simulink model "scar22"  (R2021a)
settings: Solver=ode23tb  StartTime=0.0  StopTime=.2  RelTol=1e-3
libraries: spsThreePhaseSeriesRLCLoadLib x17, spsThreePhasePISectionLineLib x16, spsThreePhaseTransformerTwoWindingsLib x14, spsThreePhaseVIMeasurementLib x11, simulink x6, exampleMicrogridLibrary x6, spsThreePhaseParallelRLCBranchLib x5, spsThreePhaseDynamicLoadLib x5, spsGroundLib x4, spsAC1AExcitationSystemLib x2, spsDieselMotorModel x2, spsSynchronousMachinepuStandardLib x2
(part 1 of 2)
settings Model: Creator=jlesage  LastModifiedBy=Administrator
settings SolverCC: AlgebraicLoopSolver=TrustRegion
settings DataIOCC: SaveFormat=Array  ReturnWorkspaceOutputs=off  DatasetSignalFormat=timetable
settings DebuggingCC: UnconnectedInputMsg=none  UnconnectedOutputMsg=none  UnconnectedLineMsg=none  SFMachineParentedDataDiag=warning  ArithmeticOperatorsInVariantConditions=warning
settings SFSimCC: SimUseLocalCustomCode=off  CustomCodeUndefinedFunction=UseInterfaceOnly
settings RTWCC: RTWUseLocalCustomCode=off

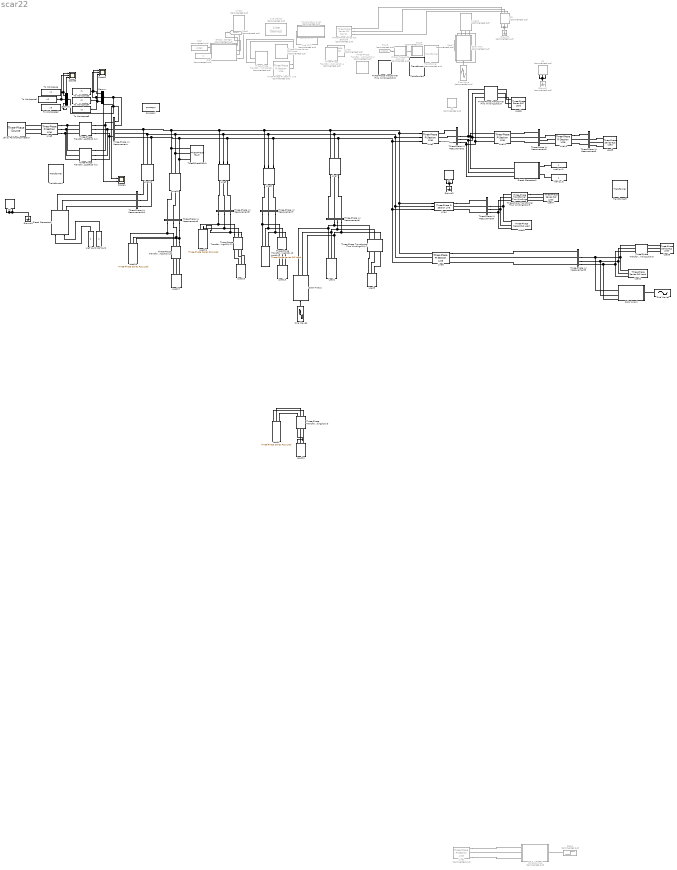
== system scar22 ==
  C1 : spsThreePhaseParallelRLCBranchLib/Three-Phase Parallel RLC Branch  Commented=on  LConnTagsString=A|B|C  RConnTagsString=A|B|C  BranchType=C  Resistance=1  Inductance=0.2e-2  Capacitance=550e-5  Measurements=None
      settings: SourceProductBaseCode=PS
  C2 : spsThreePhaseParallelRLCBranchLib/Three-Phase Parallel RLC Branch  Commented=on  LConnTagsString=A|B|C  RConnTagsString=A|B|C  BranchType=C  Resistance=1  Inductance=0.2e-2  Capacitance=550e-5  Measurements=None
      settings: SourceProductBaseCode=PS
  C3 : spsThreePhaseParallelRLCBranchLib/Three-Phase Parallel RLC Branch  Commented=on  LConnTagsString=A|B|C  RConnTagsString=A|B|C  BranchType=C  Resistance=1  Inductance=0.2e-2  Capacitance=550e-5  Measurements=None
      settings: SourceProductBaseCode=PS
  C4 : spsThreePhaseParallelRLCBranchLib/Three-Phase Parallel RLC Branch  LConnTagsString=A|B|C  RConnTagsString=A|B|C  BranchType=C  Resistance=1  Inductance=0.2e-2  Capacitance=1e6  Measurements=None
      settings: SourceProductBaseCode=PS
  C5 : spsThreePhaseParallelRLCBranchLib/Three-Phase Parallel RLC Branch  LConnTagsString=A|B|C  RConnTagsString=A|B|C  BranchType=R  Resistance=1e6  Inductance=0.2e-2  Capacitance=550e-5  Measurements=None
      settings: SourceProductBaseCode=PS
  Demux : Demux  Outputs=3
  Demux1 : Demux  Outputs=3
  Diesel Generator1 : Subsystem  mask(Diesel Generator (Simple)){Pn=3.5e6, Vn=10000, Fn=50, genType=PQ, PQ0=[0.05 0]}
      mask prompts: Pn "Generator Rated Power [W]"; Vn "Rated Voltage [V]"; Fn "Rated Frequency [Hz]"; genType "Load Flow Type"; PQ0 "Initial Power, [P0 Q0] [pu]"
      mask help:
      | The Diesel Generator block contains a synchronous generator, diesel governor and excitation system to represent the dynamics of a Genset. To inspect the model, look under the block mask (Ctrl + u).
      |
      | The inputs to the basic Diesel generator block are the desired speed reference (in pu) and the desired voltage reference (in pu). The output measurements are contained in a Simulink bus, which can be selected by using the Bus Selector block.
      |
      | Note: The initial generator power must be specified for use for Load Flow analysis.
      mask init:
      | % Extract Initial Active/Reactive Power
      | P0 = PQ0(1);
      | Q0 = PQ0(2);
      | 
      | % Select Load Flow Type
      | genBlock = [gcb '/Synchronous Machine'];
      | currentVals = get_param(genBlock,'MaskValues');
      | currentVals{31} = genType;
      | set_param(genBlock,'MaskValues',currentVals);
      | 
      | % Disable Option if Swing Generator Selected
      | currentEnables = get_param(gcb,'MaskEnables');
      | if strcmp(genType,'swing')
      |     currentEnables{5} = 'off';
      | else
      |     currentEnables{5} = 'on';
      | end
      | set_param(gcb,'MaskEnables',currentEnables);
      settings: AttributesFormatString=Rated Power: %<Pn> W
      mask TypeOptions genType: swing | PQ | PV
      mask Display: %image(imread('diesel.jpg'))
  Diesel Generator2 : Subsystem  mask(Diesel Generator (Simple)){Pn=7.6e6, Vn=10000, Fn=50, genType=PQ, PQ0=[0.05 0]}
      mask prompts: Pn "Generator Rated Power [W]"; Vn "Rated Voltage [V]"; Fn "Rated Frequency [Hz]"; genType "Load Flow Type"; PQ0 "Initial Power, [P0 Q0] [pu]"
      mask help:
      | The Diesel Generator block contains a synchronous generator, diesel governor and excitation system to represent the dynamics of a Genset. To inspect the model, look under the block mask (Ctrl + u).
      |
      | The inputs to the basic Diesel generator block are the desired speed reference (in pu) and the desired voltage reference (in pu). The output measurements are contained in a Simulink bus, which can be selected by using the Bus Selector block.
      |
      | Note: The initial generator power must be specified for use for Load Flow analysis.
      mask init: same as scar22/Diesel Generator1
      settings: AttributesFormatString=Rated Power: %<Pn> W
      mask TypeOptions genType: swing | PQ | PV
      mask Display: %image(imread('diesel.jpg'))
  Energy Storage : Subsystem  Commented=on  mask(Grid-connected Energy Storage (PQ Model)){Vn=5000, Fn=50, PnomkW=500, kWh_Rated=100, Efficiency=96, LimitVec=[90 10], RechargeSOC=11, Precharge=50, autoRecharge=off, Initial_kWh_pc=80, PQvec=[500e3 0]}
      mask prompts: Vn "Nominal L-L Voltage [Vrms]"; Fn "Nominal Frequency [Hz]"; PnomkW "Rated Power [kW]"; kWh_Rated "Rated Capacity [kWh]"; Efficiency "Overall System Efficiency [%]"; LimitVec "Upper/Lower Charge Limits [%]"; RechargeSOC "SOC to Recharge [%]"; Precharge "Recharge Rate [% of Rated Power]"; autoRecharge "Enable Auto-Recharge"; Initial_kWh_pc "Initial State-of-Charge [0-100%]"; PQvec "Initial Active/Reactive Cmds"
      mask help:
      | The energy storage block models a generic grid-connected energy storage system (ESS), most commonly a battery system. This is a system-level model that does not contain any power electronics, but is useful for load flow, phasor, and hybrid phasor-EMT simulations. The inputs to this block are the commanded active and reactive power of the ESS. The ESS is assumed to have four quadrent operation.
      |
      | For more detailed ESS models, consider the battery block in the Drives library. Consider using this PQ Model to perform load flow studies and switch to a more detailed model when full EMT studies or more advanced controls are required.
      |
      | Note: The initial active/reactive power commands must be specified for use for Load Flow analysis.
      mask init:
      | % Calculate Initial Conditions
      | Pnom = PnomkW*1e3;
      | P0 = -PQvec(1);  Q0 = -PQvec(2);
      | if abs(P0) > Pnom
      |     P0 = sign(P0)*Pnom;
      | end
      | 
      | % Calculate Q0 given Reactive Power Capability Curve
      | Qlim = sqrt(Pnom^2 - P0^2);
      | if Qlim > abs(Q0)
      |     Q0 = sign(Q0)*Qlim;
      | end
      | 
      | UpChrgLim = LimitVec(1);
      | LowChrgLim = LimitVec(2);
      | if Initial_kWh_pc > UpChrgLim && P0 < 0
      |     P0 = 0; Q0 = 0;
      | elseif Initial_kWh_pc < LowChrgLim && P0 > 0
      |     P0 = 0; Q0 = 0;
      | end
      mask DialogControl Container7 Prompt: Grid Connection Properties
      mask DialogControl Container11 Prompt: Charge/Discharge Controls
      mask DialogControl Container12 Prompt: Initial Conditions
  From3 : From  Commented=on  GotoTag=Vabc  TagVisibility=global
  Goto1 : Goto  Commented=on  GotoTag=battM  TagVisibility=global
  Goto2 : Goto  Commented=on  GotoTag=pvM  TagVisibility=global
  Ground1 : spsGroundLib/Ground  Commented=on  LConnTagsString=a
  Ground2 : spsGroundLib/Ground  LConnTagsString=a
  Ground3 : spsGroundLib/Ground  Commented=on  LConnTagsString=a
  Ground4 : spsGroundLib/Ground  LConnTagsString=a
  Line (PI)1 : exampleMicrogridLibrary/Line (PI)  Commented=on  gauge=500 Kcmil  Freq=60  Length_ft=50  Ratio=3
  Line (Series) : exampleMicrogridLibrary/Line (Series)  Commented=on  gauge=500 Kcmil  Length=50
  Line1 : spsThreePhasePISectionLineLib/Three-Phase PI Section Line  Commented=on  LConnTagsString=a|b|c  RConnTagsString=A|B|C  Length=1  Frequency=50  Resistances=[ 0.01273 0.3864]  Inductances="[ 0.9337e-3  4.1264e-3]"  Capacitances=[12.74e-9 7.751e-9]
  Line10 : spsThreePhasePISectionLineLib/Three-Phase PI Section Line  Commented=on  LConnTagsString=a|b|c  RConnTagsString=A|B|C  Length=1  Frequency=50  Resistances="[ 0.206  0.96 ]"  Inductances="[ 0.359e-3   1.178e-3 ]"  Capacitances="[0.254e-6  0.118e-6 ]"
  Line11 : spsThreePhasePISectionLineLib/Three-Phase PI Section Line  Commented=on  LConnTagsString=a|b|c  RConnTagsString=A|B|C  Length=1  Frequency=50  Resistances="[ 0.206  0.96 ]"  Inductances="[ 0.359e-3   1.178e-3 ]"  Capacitances="[0.254e-6  0.118e-6 ]"
  Line{2,4,6..9,12..15} (10 alike) : spsThreePhasePISectionLineLib/Three-Phase PI Section Line  LConnTagsString=a|b|c  RConnTagsString=A|B|C  Length=1  Frequency=50  Resistances="[ 0.206  0.96 ]"  Inductances="[ 0.359e-3   1.178e-3 ]"  Capacitances="[0.254e-6  0.118e-6 ]"
  Line3 : spsThreePhasePISectionLineLib/Three-Phase PI Section Line  Commented=on  LConnTagsString=a|b|c  RConnTagsString=A|B|C  Length=1  Frequency=50  Resistances="[ 0.206  0.96 ]"  Inductances="[ 0.359e-3   1.178e-3 ]"  Capacitances="[0.254e-6  0.118e-6 ]"
  Line5 : spsThreePhasePISectionLineLib/Three-Phase PI Section Line  LConnTagsString=a|b|c  RConnTagsString=A|B|C  Length=1  Frequency=50  Resistances=[ 0.01273 0.3864]  Inductances="[ 0.9337e-3  4.1264e-3]"  Capacitances=[12.74e-9 7.751e-9]
  Load{1..5,14,16,18} (8 alike) : spsThreePhaseSeriesRLCLoadLib/Three-Phase Series RLC Load  LConnTagsString=A|B|C  Configuration=Y (grounded)  NominalVoltage=10000  Vabc=[1e3 1e3 1e3]  Vabcp=[1e3 1e3 1e3]  NominalFrequency=50  UnbalancedPower=off  ActivePower=500e3  InductivePower=0  CapacitivePower=0  Pabc=[10e3 9e3 11e3]  QLabc=[100 90 110]  QCabc=[100 90 110]  Pabcp=[10e3 9e3 11e3]  QLabcp=[100 90 110]  QCabcp=[100 90 110]  Measurements=None  LoadType=constant Z
      settings: AttributesFormatString=P = %<ActivePower> W
  Load{6..10,13,15,17} (8 alike) : spsThreePhaseSeriesRLCLoadLib/Three-Phase Series RLC Load  LConnTagsString=A|B|C  Configuration=Y (grounded)  NominalVoltage=400  Vabc=[1e3 1e3 1e3]  Vabcp=[1e3 1e3 1e3]  NominalFrequency=50  UnbalancedPower=off  ActivePower=500e3  InductivePower=0  CapacitivePower=0  Pabc=[10e3 9e3 11e3]  QLabc=[100 90 110]  QCabc=[100 90 110]  Pabcp=[10e3 9e3 11e3]  QLabcp=[100 90 110]  QCabcp=[100 90 110]  Measurements=None  LoadType=constant Z
      settings: AttributesFormatString=P = %<ActivePower> W
  Phasor Sequence Analyzer : Subsystem  Commented=on
  Pref : Constant  Commented=on  Value=100e3
  Qref : Constant  Commented=on  Value=0
  Scope : Subsystem  Commented=on
  Scope1 : Scope  NumInputPorts=2
  Scope2 : Scope  NumInputPorts=3
  Scope3 : Scope  NumInputPorts=3
  Sine Wave : Sin  Commented=on  Amplitude=200e3  Bias=250e3  Frequency=0.05  SampleTime=0
  Sine Wave1 : Sin  Amplitude=200e3  Bias=250e3  Frequency=0.05  SampleTime=0
  Sine Wave2 : Sin  Amplitude=200e3  Bias=250e3  Frequency=0.05  SampleTime=0
  Solar Array : Subsystem  Commented=on  mask(Grid-Connected PV Array (PQ Model)){Vn=5000, Fn=50, P0=500e3}
      mask prompts: Vn "Nominal L-L Voltage [Vrms]"; Fn "Nominal Frequency [Hz]"; P0 "Initial Power [W]"
      mask help:
      | This block models a grid-connected solar array using the Three-Phase Dynamic Load block. This is a system-level model that does not contain any power electronics, but is useful for load flow, phasor, and hybrid phasor-EMT simulations. The input to this block is the power output of the grid connected PV array, not irradiance.
      |
      | For more detailed PV models, consider the PV Array block in the Renewables library. Consider using this PQ Model to perform load flow studies and switch to a more detailed model when full EMT studies are required.
      |
      | Note: The array power must be specified for use for Load Flow analysis.
      mask init:
      | % P0 = Irr0*TotalArea*Efficiency/100;
      | P0 = -P0;
      mask Display:
      | image(imread('PV_Farm.jpg'))
      | color('white')
      | port_label('input',1,'P')
      | port_label('output',1,'m')
      | port_label('Rconn',1,'A')
      | port_label('Rconn',2,'B')
      | port_label('Rconn',3,'C')
  Solar Array1 : Subsystem  mask(Grid-Connected PV Array (PQ Model)){Vn=10000, Fn=50, P0=500e3}
      mask prompts: Vn "Nominal L-L Voltage [Vrms]"; Fn "Nominal Frequency [Hz]"; P0 "Initial Power [W]"
      mask help:
      | This block models a grid-connected solar array using the Three-Phase Dynamic Load block. This is a system-level model that does not contain any power electronics, but is useful for load flow, phasor, and hybrid phasor-EMT simulations. The input to this block is the power output of the grid connected PV array, not irradiance.
      |
      | For more detailed PV models, consider the PV Array block in the Renewables library. Consider using this PQ Model to perform load flow studies and switch to a more detailed model when full EMT studies are required.
      |
      | Note: The array power must be specified for use for Load Flow analysis.
      mask init:
      | % P0 = Irr0*TotalArea*Efficiency/100;
      | P0 = -P0;
      mask Display:
      | image(imread('PV_Farm.jpg'))
      | color('white')
      | port_label('input',1,'P')
      | port_label('output',1,'m')
      | port_label('Rconn',1,'A')
      | port_label('Rconn',2,'B')
      | port_label('Rconn',3,'C')
  Solar Array2 : Subsystem  mask(Grid-Connected PV Array (PQ Model)){Vn=10000, Fn=50, P0=500e3}
      mask prompts: Vn "Nominal L-L Voltage [Vrms]"; Fn "Nominal Frequency [Hz]"; P0 "Initial Power [W]"
      mask help:
      | This block models a grid-connected solar array using the Three-Phase Dynamic Load block. This is a system-level model that does not contain any power electronics, but is useful for load flow, phasor, and hybrid phasor-EMT simulations. The input to this block is the power output of the grid connected PV array, not irradiance.
      |
      | For more detailed PV models, consider the PV Array block in the Renewables library. Consider using this PQ Model to perform load flow studies and switch to a more detailed model when full EMT studies are required.
      |
      | Note: The array power must be specified for use for Load Flow analysis.
      mask init:
      | % P0 = Irr0*TotalArea*Efficiency/100;
      | P0 = -P0;
      mask Display:
      | image(imread('PV_Farm.jpg'))
      | color('white')
      | port_label('input',1,'P')
      | port_label('output',1,'m')
      | port_label('Rconn',1,'A')
      | port_label('Rconn',2,'B')
      | port_label('Rconn',3,'C')
  Step2 : Step  Commented=on  Time=35  Before=200e3  After=500e3  SampleTime=0
  Three-Phase PI Section Line : spsThreePhasePISectionLineLib/Three-Phase PI Section Line  Commented=on  LConnTagsString=a|b|c  RConnTagsString=A|B|C  Length=10  Frequency=50  Resistances=[ 0.01273 0.3864]  Inductances="[ 0.9337e-3  4.1264e-3]"  Capacitances=[12.74e-9 7.751e-9]
  Three-Phase Series RLC Branch8 : spsThreePhaseSeriesRLCBranchLib/Three-Phase Series RLC Branch  Commented=on  LConnTagsString=A|B|C  RConnTagsString=A|B|C  BranchType=RL  Resistance=.15*3  Inductance=1.3263e-3*3  Capacitance=1e-6  Measurements=None
  Three-Phase Series RLC Load : spsThreePhaseSeriesRLCLoadLib/Three-Phase Series RLC Load  Commented=on  LConnTagsString=A|B|C  Configuration=Y (grounded)  NominalVoltage=1000  Vabc=[1e3 1e3 1e3]  Vabcp=[1e3 1e3 1e3]  NominalFrequency=60  UnbalancedPower=off  ActivePower=10e3  InductivePower=100  CapacitivePower=100  Pabc=[10e3 9e3 11e3]  QLabc=[100 90 110]  QCabc=[100 90 110]  Pabcp=[10e3 9e3 11e3]  QLabcp=[100 90 110]  QCabcp=[100 90 110]  Measurements=None  LoadType=constant Z
  Three-Phase Transformer (Two Windings)10/.1 : spsThreePhaseTransformerTwoWindingsLib/Three-Phase Transformer (Two Windings)  Commented=on  Winding1Connection=Yg  Winding2Connection=Yg  CoreType=Three single-phase transformers  SetSaturation=off  Hysteresis=off  DataFile='hysteresis'  SetInitialFlux=off  Measurements=None  UNITS=pu  NominalPower=[ 360000 , 50]  Winding1=[ 10e3 , 9.075313e-4 , 1.77250502e-7]  Winding2=[ 400 , 3.023598725e-4 , 5.906247735e-8]  Rm=500  Lm=500  L0=0.5  Saturation=[ 0,0 ; 0.0024,1.2 ; 1.0,1.52 ]  InitialFluxes=[ 0.8 , -0.8 , 0.7 ]  BreakLoop=off  DiscreteSolver=Trapezoidal iterative  DataType=off  TransfoNumber=1
  Three-Phase Transformer (Two Windings)10/.{3,5..12} (9 alike) : spsThreePhaseTransformerTwoWindingsLib/Three-Phase Transformer (Two Windings)  Winding1Connection=Yg  Winding2Connection=Yg  CoreType=Three single-phase transformers  SetSaturation=off  Hysteresis=off  DataFile='hysteresis'  SetInitialFlux=off  Measurements=None  UNITS=pu  NominalPower=[ 360000 , 50]  Winding1=[ 10e3 , 9.075313e-4 , 1.77250502e-7]  Winding2=[ 400 , 3.023598725e-4 , 5.906247735e-8]  Rm=500  Lm=500  L0=0.5  Saturation=[ 0,0 ; 0.0024,1.2 ; 1.0,1.52 ]  InitialFluxes=[ 0.8 , -0.8 , 0.7 ]  BreakLoop=off  DiscreteSolver=Trapezoidal iterative  DataType=off  TransfoNumber=1
  Three-Phase Transformer (Two Windings)10/.2 : spsThreePhaseTransformerTwoWindingsLib/Three-Phase Transformer (Two Windings)  Commented=on  Winding1Connection=Yg  Winding2Connection=Yg  CoreType=Three single-phase transformers  SetSaturation=off  Hysteresis=off  DataFile='hysteresis'  SetInitialFlux=off  Measurements=None  UNITS=pu  NominalPower=[ 360000 , 50]  Winding1=[ 10e3 , 9.075313e-4 , 1.77250502e-7]  Winding2=[ 400 , 3.023598725e-4 , 5.906247735e-8]  Rm=500  Lm=500  L0=0.5  Saturation=[ 0,0 ; 0.0024,1.2 ; 1.0,1.52 ]  InitialFluxes=[ 0.8 , -0.8 , 0.7 ]  BreakLoop=off  DiscreteSolver=Trapezoidal iterative  DataType=off  TransfoNumber=1
  Three-Phase Transformer (Two Windings)10/.4 : spsThreePhaseTransformerTwoWindingsLib/Three-Phase Transformer (Two Windings)  Commented=on  Winding1Connection=Yg  Winding2Connection=Yg  CoreType=Three single-phase transformers  SetSaturation=off  Hysteresis=off  DataFile='hysteresis'  SetInitialFlux=off  Measurements=None  UNITS=pu  NominalPower=[ 360000 , 50]  Winding1=[ 10e3 , 9.075313e-4 , 1.77250502e-7]  Winding2=[ 400 , 3.023598725e-4 , 5.906247735e-8]  Rm=500  Lm=500  L0=0.5  Saturation=[ 0,0 ; 0.0024,1.2 ; 1.0,1.52 ]  InitialFluxes=[ 0.8 , -0.8 , 0.7 ]  BreakLoop=off  DiscreteSolver=Trapezoidal iterative  DataType=off  TransfoNumber=1
  Three-Phase Transformer (Two Windings)35/10 kv1 : spsThreePhaseTransformerTwoWindingsLib/Three-Phase Transformer (Two Windings)  Winding1Connection=Yg  Winding2Connection=Yg  CoreType=Three single-phase transformers  SetSaturation=off  Hysteresis=off  DataFile='hysteresis'  SetInitialFlux=off  Measurements=None  UNITS=pu  NominalPower=[ 8e6 , 50]  Winding1=[ 35e3 , 3.023998286e-4 , 1.518786171e-6]  Winding2=[ 10000 , 9.07159816e-4 , 4.566281711e-6]  Rm=500  Lm=500  L0=0.5  Saturation=[ 0,0 ; 0.0024,1.2 ; 1.0,1.52 ]  InitialFluxes=[ 0.8 , -0.8 , 0.7 ]  BreakLoop=off  DiscreteSolver=Trapezoidal iterative  DataType=off  TransfoNumber=1
  Three-Phase Transformer (Two Windings)35/10 kv2 : spsThreePhaseTransformerTwoWindingsLib/Three-Phase Transformer (Two Windings)  Winding1Connection=Yg  Winding2Connection=Yg  CoreType=Three single-phase transformers  SetSaturation=off  Hysteresis=off  DataFile='hysteresis'  SetInitialFlux=off  Measurements=None  UNITS=pu  NominalPower=[ 8e6 , 50]  Winding1=[ 35e3 , 3.023998286e-4 , 1.518786171e-6]  Winding2=[ 10000 , 9.07159816e-4 , 4.566281711e-6]  Rm=500  Lm=500  L0=0.5  Saturation=[ 0,0 ; 0.0024,1.2 ; 1.0,1.52 ]  InitialFluxes=[ 0.8 , -0.8 , 0.7 ]  BreakLoop=off  DiscreteSolver=Trapezoidal iterative  DataType=off  TransfoNumber=1
  Three-Phase V-I Measurement{,1..6} (7 alike) : spsThreePhaseVIMeasurementLib/Three-Phase V-I Measurement  VoltageMeasurement=phase-to-ground  SetLabelV=off  LabelV=Vabc  Vpu=off  VpuLL=off  CurrentMeasurement=yes  SetLabelI=off  LabelI=Iabc  Ipu=off  Pbase=100e6  Vbase=500e3  OutputType=Complex  PhasorSimulation=off  PSBequivalent=0
  Three-Phase V-I Measurement{7..10} (4 alike) : spsThreePhaseVIMeasurementLib/Three-Phase V-I Measurement  VoltageMeasurement=no  SetLabelV=off  LabelV=Vabc  Vpu=off  VpuLL=off  CurrentMeasurement=no  SetLabelI=off  LabelI=Iabc  Ipu=off  Pbase=100e6  Vbase=500e3  OutputType=Complex  PhasorSimulation=off  PSBequivalent=0
  Three-Phase Fault : spsThreePhaseFaultLib/Three-Phase Fault  InitialStates=0  FaultA=on  FaultB=on  FaultC=off  GroundFault=on  SwitchTimes="[.07   ]"  External=off  SwitchStatus=NaN  FaultResistance=0.001  GroundResistance=0.01  SnubberResistance=1e6  SnubberCapacitance=inf  Measurements=None
  To Workspace : ToWorkspace  VariableName=v1  SampleTime=-1
  To Workspace1 : ToWorkspace  VariableName=v2  SampleTime=-1
  To Workspace2 : ToWorkspace  VariableName=v3  SampleTime=-1
  To Workspace3 : ToWorkspace  VariableName=i1  SampleTime=-1
  To Workspace4 : ToWorkspace  VariableName=i2  SampleTime=-1
  To Workspace5 : ToWorkspace  VariableName=i3  SampleTime=-1
  Transformer : exampleMicrogridLibrary/Transformer  Commented=on  kS=225  Freq=60  Vp=4160  Vs=460  Zperc=5.18  Ratio=2.5
  Transformer1 : exampleMicrogridLibrary/Transformer  kS=225  Freq=50  Vp=10000  Vs=6300  Zperc=5.18  Ratio=2.5
  Transformer3 : exampleMicrogridLibrary/Transformer  kS=225  Freq=50  Vp=10000  Vs=6300  Zperc=5.18  Ratio=2.5
  Transformer4 : exampleMicrogridLibrary/Transformer  kS=225  Freq=50  Vp=10000  Vs=6300  Zperc=5.18  Ratio=2.5
  Transmission Line1 : Subsystem  Commented=on  mask(Transmission Line Short Line Model){f=60, LineProperty=Resistance and Inductance, R=0.15, L=0.0013263, Z=0.15+0.5i, Length=40}
      mask prompts: f "Line Frequency (Hz)"; LineProperty "Line Electrical Property in"; R "Resistance Per Unit Length (Ohms/km)"; L "Inductance Per Unit Length (H/km)"; Z "Impedance Per Unit Length (R+Li/km)"; Length "Line Length (km)"
      mask help:
      | Transmission Line Short Line Model developed by Dr Rodney Tan
      | Version 1.0 (Oct 2017)
      |
      | Transmission line short line model block is compute using three phase series RL branch based on its line length (km), resistance per unit length (Ohms/km), inductance per unit length (H/km) or Impedance per unit length (R+Li/km) in complex number.
      mask TypeOptions f: 50 | 60
      mask TypeOptions LineProperty: Resistance and Inductance | Impedance
      mask Callback LineProperty:
      | switch(get_param(gcb,'LineProperty'))
      |     case 'Resistance and Inductance'
      |         set_param(gcb,'MaskEnables',{'on','on','on','on','off','on'});
      |     otherwise
      |         set_param(gcb,'MaskEnables',{'on','on','off','off','on','on'});
      | end
      mask Callback R:
      | R = str2double(get_param(gcb,'R'));
      | L = str2double(get_param(gcb,'L'));
      | f = str2double(get_param(gcb,'f'));
      | set_param(gcb,'Z',num2str(complex(R,2*pi*f*L)));
      mask Callback L:
      | R = str2double(get_param(gcb,'R'));
      | L = str2double(get_param(gcb,'L'));
      | f = str2double(get_param(gcb,'f'));
      | set_param(gcb,'Z',num2str(complex(R,2*pi*f*L)));
      mask Callback Z:
      | Z = str2double(get_param(gcb,'Z'));
      | if ~any(imag(Z))||isnan(Z)
      |     msgbox('Line Impedance must be in Complex Number',...
      |     'Invalid Value !','error');
      |     set_param(gcb,'Z','0.15+0.5i');
      |     return
      | end
      | f = str2double(get_param(gcb,'f'));
      | set_param(gcb,'R',num2str(real(Z)));
      | set_param(gcb,'L',num2str(imag(Z)/(2*pi*f)));
      mask Callback Length:
      | Length = str2double(get_param(gcb,'Length'));
      | if (Length > 100)||(Length < 0.1)||isnan(Length)
      |     msgbox('Line Length must be in the range of 0.1-100',...
      |     'Invalid Value !','error');
      |     set_param(gcb,'Length','40');
      | end
      mask Display:
      | disp('Short Line Model');
      | port_label('lconn',1,'A');
      | port_label('lconn',2,'B');
      | port_label('lconn',3,'C');
      | port_label('rconn',1,'a');
      | port_label('rconn',2,'b');
      | port_label('rconn',3,'c');
  Utility Point-of-Connection : spsThreePhaseSourceLib/Three-Phase Source  InternalConnection=Yg  VoltagePhases=off  Voltage=(13800)*1.00243  PhaseAngle=0.071468  Voltage_phases=[25e3 25e3 25e3]/sqrt(3)  PhaseAngles_phases=[0 -120 +120]  Frequency=50  NonIdealSource=on  SpecifyImpedance=on  Resistance=0.8929  Inductance=16.58e-3  ShortCircuitLevel=250e6  BaseVoltage=13.8e3  XRratio=7  BusType=swing  Pref=10e3  Qref=0  Prefabc=[10e3, 10e3, 10e3]  Qrefabc=[0, 0, 0]  Qmin=-inf  Qmax=inf
  Variable Load : Subsystem  Commented=on  mask(Variable Load (PQ Model)){Vn=5000, Fn=50, PF=1, Load0=200e3}
      mask prompts: Vn "Nominal L-L Voltage [Vrms]"; Fn "Nominal Frequency [Hz]"; PF "Power Factor [0 to 1]"; Load0 "Initial Load [W]"
      mask help:
      | The Variable Load block is a lumped approximation for a distribution feeder. For non-unity power factor loads, the input (active power) is scaled accordingly to generate a desired load.
      |
      | Note: The initial input load must be specified for use for Load Flow analysis.
      mask init:
      | P0 = Load0;
      | Q0 = Load0*sqrt(1/PF-1);
      mask Display:
      | image(imread('Residential.jpg'))
      | color('white')
      | port_label('input',1,'Load')
      | port_label('Rconn',1,'A')
      | port_label('Rconn',2,'B')
      | port_label('Rconn',3,'C')
  Vref (pu)1 : Constant
  Vref (pu)2 : Constant
  powergui : spspowerguiLib/powergui  Priority=1  SimulationMode=Discrete  SampleTime=2.5e-5  frequency=50  Iterations=50  frequencyindice=50  Pbase=100e6  ErrMax=0.0001  UnitsV=kV  UnitsW=MW  buscounter=3  FunctionMessages=off  echomessages=off  EnableUseOfTLC=off  CurrentSourceSwitches=off  DisableSnubberDevices=off  DisableRonSwitches=off  DisableVfSwitches=off  DisplayEquations=off  AutomaticDiscreteSolvers=off  SolverType=Tustin/Backward Euler (TBE)  Interpol=off  ExternalGateDelay=off  methode=off  Ts=100  x0status=blocks  SPID=on  SwTol=0  HookPort=off  NonlinearTolerance=1e-4  nMaxIteration=100  ContinueOnMaxIteration=off  RestoreLinks=warning  ResistiveCurrentMeasurement=off  Frange=[0:2:500]  Ylog=off  Xlog=on  ShowGrid=off  save=off  variable=ZData  structure=0  ZoomFFT=off  StartTime=0.0  cycles=1  DisplayStyle=1  fundamental=60  FreqAxis=off  MaxFrequency=1000  frequencyindicesteady=1  RmsSteady=1  display=off
  wref (pu)1 : Constant
  wref (pu)2 : Constant
  wires:
  Sine Wave/1 -> Solar Array/1(P)
  Pref/1 -> Energy Storage/1(Pref)
  Qref/1 -> Energy Storage/2(Qref)
  Energy Storage/1(m) -> Goto1/1
  Step2/1 -> Variable Load/1(Load)
  Solar Array/1(m) -> Goto2/1
  Phasor Sequence Analyzer/1(Vrms) -> Scope/1(Vrms)
  From3/1 -> Phasor Sequence Analyzer/1(Vabc)
  Three-Phase V-I Measurement/1 -> Demux1/1, Scope1/1
  Three-Phase V-I Measurement/2 -> Demux/1, Scope1/2
  Demux/1 -> Scope2/1, To Workspace3/1
  Demux/2 -> Scope2/2, To Workspace4/1
  Demux/3 -> Scope2/3, To Workspace5/1
  Demux1/1 -> Scope3/1, To Workspace/1
  Demux1/2 -> Scope3/2, To Workspace1/1
  Demux1/3 -> Scope3/3, To Workspace2/1
  Sine Wave1/1 -> Solar Array1/1(P)
  Sine Wave2/1 -> Solar Array2/1(P)
  Vref (pu)1/1 -> Diesel Generator1/2(Vref (pu))
  wref (pu)1/1 -> Diesel Generator1/1(wref (pu))
  Vref (pu)2/1 -> Diesel Generator2/2(Vref (pu))
  wref (pu)2/1 -> Diesel Generator2/1(wref (pu))
  connections:
  Line5/LConn1 -- Utility Point-of-Connection/RConn1
  Line5/LConn2 -- Utility Point-of-Connection/RConn2
  Line5/LConn3 -- Utility Point-of-Connection/RConn3
  Three-Phase Transformer (Two Windings)35/10 kv1/RConn1 -- Three-Phase V-I Measurement/LConn1 -- Three-Phase Transformer (Two Windings)35/10 kv2/RConn1
  Three-Phase Transformer (Two Windings)35/10 kv1/RConn2 -- Three-Phase Transformer (Two Windings)35/10 kv2/RConn2 -- Three-Phase V-I Measurement/LConn2
  Three-Phase Transformer (Two Windings)35/10 kv1/RConn3 -- Three-Phase Transformer (Two Windings)35/10 kv2/RConn3 -- Three-Phase V-I Measurement/LConn3
  Line5/RConn1 -- Three-Phase Transformer (Two Windings)35/10 kv2/LConn1 -- Three-Phase Transformer (Two Windings)35/10 kv1/LConn1
  Line5/RConn2 -- Three-Phase Transformer (Two Windings)35/10 kv2/LConn2 -- Three-Phase Transformer (Two Windings)35/10 kv1/LConn2
  Line5/RConn3 -- Three-Phase Transformer (Two Windings)35/10 kv2/LConn3 -- Three-Phase Transformer (Two Windings)35/10 kv1/LConn3
  Variable Load/RConn2 -- Line1/RConn2
  Line1/RConn1 -- Variable Load/RConn1
  Line1/RConn3 -- Variable Load/RConn3
  Line10/RConn1 -- Solar Array/RConn1
  Line10/RConn2 -- Solar Array/RConn2
  Line10/RConn3 -- Solar Array/RConn3
  Three-Phase V-I Measurement5/LConn2 -- Line6/RConn2
  Three-Phase V-I Measurement5/LConn3 -- Line6/RConn3
  Three-Phase V-I Measurement1/LConn1 -- Line2/RConn1
  Three-Phase V-I Measurement1/LConn2 -- Line2/RConn2
  Three-Phase V-I Measurement1/LConn3 -- Line2/RConn3
  Ground3/LConn1 -- C3/RConn2 -- C3/RConn1 -- C3/RConn3
  Three-Phase Series RLC Branch8/RConn1 -- C3/LConn1
  Three-Phase Series RLC Branch8/RConn2 -- C3/LConn2
  Three-Phase Series RLC Branch8/RConn3 -- C3/LConn3
  Energy Storage/RConn3 -- Line11/RConn3
  Energy Storage/RConn2 -- Line11/RConn2
  Energy Storage/RConn1 -- Line11/RConn1
  Line2/LConn1 -- Line6/LConn1 -- Line4/LConn1 -- Line8/LConn1 -- Line9/LConn1 -- Line15/LConn1 -- Three-Phase Fault/LConn1 -- Three-Phase V-I Measurement/RConn1 -- Line14/LConn1 -- Line7/LConn1
  Line2/LConn2 -- Line7/LConn2 -- Line8/LConn2 -- Line9/LConn2 -- Three-Phase Fault/LConn2 -- Line15/LConn2 -- Three-Phase V-I Measurement/RConn2 -- Line14/LConn2 -- Line6/LConn2 -- Line4/LConn2
  Line2/LConn3 -- Line7/LConn3 -- Line8/LConn3 -- Line9/LConn3 -- Three-Phase Fault/LConn3 -- Line15/LConn3 -- Line14/LConn3 -- Three-Phase V-I Measurement/RConn3 -- Line6/LConn3 -- Line4/LConn3
  Three-Phase V-I Measurement1/RConn1 -- Three-Phase Transformer (Two Windings)10/.9/LConn1 -- Diesel Generator1/RConn1 -- Line12/LConn1
  Three-Phase V-I Measurement1/RConn2 -- Diesel Generator1/RConn2 -- Three-Phase Transformer (Two Windings)10/.9/LConn2 -- Line12/LConn2
  Three-Phase V-I Measurement1/RConn3 -- Diesel Generator1/RConn3 -- Three-Phase Transformer (Two Windings)10/.9/LConn3 -- Line12/LConn3
  Three-Phase V-I Measurement2/LConn2 -- Line12/RConn2
  Three-Phase V-I Measurement2/LConn3 -- Line12/RConn3
  Three-Phase V-I Measurement2/LConn1 -- Line12/RConn1
  Line13/LConn1 -- Three-Phase V-I Measurement2/RConn1
  Line13/LConn2 -- Three-Phase V-I Measurement2/RConn2
  Line13/LConn3 -- Three-Phase V-I Measurement2/RConn3
  Line13/RConn1 -- Three-Phase V-I Measurement3/LConn1
  Three-Phase V-I Measurement3/LConn2 -- Line13/RConn2
  Three-Phase V-I Measurement3/LConn3 -- Line13/RConn3
  Load5/LConn1 -- Three-Phase V-I Measurement3/RConn1
  Load5/LConn2 -- Three-Phase V-I Measurement3/RConn2
  Load5/LConn3 -- Three-Phase V-I Measurement3/RConn3
  Load6/LConn2 -- Three-Phase Transformer (Two Windings)10/.9/RConn2
  Load6/LConn1 -- Three-Phase Transformer (Two Windings)10/.9/RConn1
  Load6/LConn3 -- Three-Phase Transformer (Two Windings)10/.9/RConn3
  Load7/LConn2 -- Three-Phase Transformer (Two Windings)10/.5/RConn2
  Load7/LConn3 -- Three-Phase Transformer (Two Windings)10/.5/RConn3
  Three-Phase Transformer (Two Windings)10/.5/RConn1 -- Load7/LConn1
  Line4/RConn1 -- Three-Phase V-I Measurement4/LConn1
  Three-Phase V-I Measurement4/LConn2 -- Line4/RConn2
  Three-Phase V-I Measurement4/LConn3 -- Line4/RConn3
  Three-Phase V-I Measurement4/RConn1 -- Load3/LConn1 -- Three-Phase Transformer (Two Windings)10/.5/LConn1
  Three-Phase V-I Measurement4/RConn2 -- Load3/LConn2 -- Three-Phase Transformer (Two Windings)10/.5/LConn2
  Three-Phase V-I Measurement4/RConn3 -- Load3/LConn3 -- Three-Phase Transformer (Two Windings)10/.5/LConn3
  Load2/LConn1 -- Three-Phase V-I Measurement5/RConn1 -- Solar Array1/RConn1 -- Three-Phase Transformer (Two Windings)10/.6/LConn1
  Load2/LConn2 -- Three-Phase V-I Measurement5/RConn2 -- Solar Array1/RConn2 -- Three-Phase Transformer (Two Windings)10/.6/LConn2
  Load2/LConn3 -- Three-Phase V-I Measurement5/RConn3 -- Solar Array1/RConn3 -- Three-Phase Transformer (Two Windings)10/.6/LConn3
  Load8/LConn3 -- Three-Phase Transformer (Two Windings)10/.6/RConn3
  Line6/RConn1 -- Three-Phase V-I Measurement5/LConn1
  Load8/LConn2 -- Three-Phase Transformer (Two Windings)10/.6/RConn2
  Load8/LConn1 -- Three-Phase Transformer (Two Windings)10/.6/RConn1
  Load9/LConn1 -- Three-Phase Transformer (Two Windings)10/.7/RConn1
  Line7/RConn1 -- Three-Phase V-I Measurement6/LConn1
  Load9/LConn2 -- Three-Phase Transformer (Two Windings)10/.7/RConn2
  Load9/LConn3 -- Three-Phase Transformer (Two Windings)10/.7/RConn3
  Line7/RConn2 -- Three-Phase V-I Measurement6/LConn2
  Line7/RConn3 -- Three-Phase V-I Measurement6/LConn3
  Three-Phase PI Section Line/RConn1 -- Three-Phase Transformer (Two Windings)10/.1/LConn2
  Three-Phase PI Section Line/RConn2 -- Three-Phase Transformer (Two Windings)10/.1/LConn3
  Load4/LConn1 -- Three-Phase Transformer (Two Windings)10/.3/LConn1
  Load4/LConn2 -- Three-Phase Transformer (Two Windings)10/.3/LConn2
  Load4/LConn3 -- Three-Phase Transformer (Two Windings)10/.3/LConn3
  Load10/LConn3 -- Three-Phase Transformer (Two Windings)10/.3/RConn3
  Load10/LConn1 -- Three-Phase Transformer (Two Windings)10/.3/RConn1
  Load10/LConn2 -- Three-Phase Transformer (Two Windings)10/.3/RConn2
  Load14/LConn1 -- Three-Phase Transformer (Two Windings)10/.10/LConn1 -- Three-Phase V-I Measurement7/RConn1
  Load14/LConn2 -- Three-Phase Transformer (Two Windings)10/.10/LConn2 -- Three-Phase V-I Measurement7/RConn2
  Load14/LConn3 -- Three-Phase Transformer (Two Windings)10/.10/LConn3 -- Three-Phase V-I Measurement7/RConn3
  Load13/LConn1 -- Three-Phase Transformer (Two Windings)10/.10/RConn1
  Load13/LConn3 -- Three-Phase Transformer (Two Windings)10/.10/RConn3
  Load13/LConn2 -- Three-Phase Transformer (Two Windings)10/.10/RConn2
  Line8/RConn1 -- Three-Phase V-I Measurement7/LConn1
  Three-Phase V-I Measurement7/LConn2 -- Line8/RConn2
  Three-Phase V-I Measurement7/LConn3 -- Line8/RConn3
  Three-Phase Transformer (Two Windings)10/.11/LConn1 -- Load16/LConn1 -- Three-Phase V-I Measurement8/RConn1
  Three-Phase Transformer (Two Windings)10/.11/LConn2 -- Load16/LConn2 -- Three-Phase V-I Measurement8/RConn2
  Three-Phase Transformer (Two Windings)10/.11/LConn3 -- Load16/LConn3 -- Three-Phase V-I Measurement8/RConn3
  Load15/LConn2 -- Three-Phase Transformer (Two Windings)10/.11/RConn2
  Load15/LConn3 -- Three-Phase Transformer (Two Windings)10/.11/RConn3
  Load15/LConn1 -- Three-Phase Transformer (Two Windings)10/.11/RConn1
  Three-Phase V-I Measurement8/LConn1 -- Line9/RConn1
  Three-Phase V-I Measurement8/LConn2 -- Line9/RConn2
  Three-Phase V-I Measurement8/LConn3 -- Line9/RConn3
  Load18/LConn1 -- Three-Phase Transformer (Two Windings)10/.12/LConn1 -- Three-Phase V-I Measurement9/RConn1
  Load18/LConn2 -- Three-Phase Transformer (Two Windings)10/.12/LConn2 -- Three-Phase V-I Measurement9/RConn2
  Load18/LConn3 -- Three-Phase Transformer (Two Windings)10/.12/LConn3 -- Three-Phase V-I Measurement9/RConn3
  Three-Phase V-I Measurement9/LConn3 -- Line15/RConn3
  Three-Phase V-I Measurement9/LConn1 -- Line15/RConn1
  Load17/LConn1 -- Three-Phase Transformer (Two Windings)10/.12/RConn1
  Load17/LConn2 -- Three-Phase Transformer (Two Windings)10/.12/RConn2
  Three-Phase V-I Measurement9/LConn2 -- Line15/RConn2
  Load17/LConn3 -- Three-Phase Transformer (Two Windings)10/.12/RConn3
  Three-Phase V-I Measurement10/LConn1 -- Line14/RConn1
  Three-Phase V-I Measurement10/LConn2 -- Line14/RConn2
  Three-Phase V-I Measurement10/LConn3 -- Line14/RConn3
  Diesel Generator2/RConn1 -- Three-Phase V-I Measurement10/RConn1
  Diesel Generator2/RConn2 -- Three-Phase V-I Measurement10/RConn2
  Diesel Generator2/RConn3 -- Three-Phase V-I Measurement10/RConn3
  Load1/LConn1 -- Three-Phase V-I Measurement6/RConn1 -- Three-Phase Transformer (Two Windings)10/.7/LConn1 -- Solar Array2/RConn1
  Load1/LConn2 -- Three-Phase V-I Measurement6/RConn2 -- Three-Phase Transformer (Two Windings)10/.7/LConn2 -- Solar Array2/RConn2
  Load1/LConn3 -- Solar Array2/RConn3 -- Three-Phase V-I Measurement6/RConn3 -- Three-Phase Transformer (Two Windings)10/.7/LConn3
  Transformer1/RConn1 -- Transformer/LConn3
  C2/RConn2 -- C2/RConn3 -- C2/RConn1 -- Ground1/LConn1
  C4/RConn3 -- C4/RConn2 -- Ground2/LConn1 -- C4/RConn1
  C5/RConn2 -- C5/RConn3 -- Ground4/LConn1 -- C5/RConn1

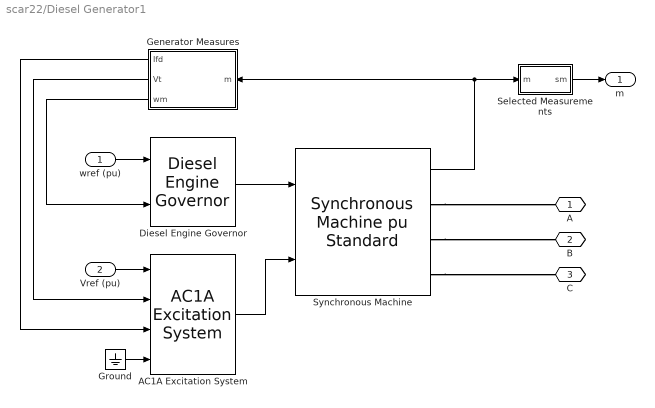
== system scar22/Diesel Generator1 ==
  wref (pu) : Inport
  Vref (pu) : Inport  Port=2
  AC1A Excitation System : spsAC1AExcitationSystemLib/AC1A Excitation System  Tr=20e-3  KaTa=[400 0.02]  VAminmax=[-14.5 14.5]  VRminmax=[-5.43 6.03]  KfTf=[0.03 1.0]  TbTc=[0 0]  KeTe=[1.0 0.80]  Ve12=[4.18 3.14]  SeVe12=[0.10 0.03]  Kd=0.38  Kc=0.20  v0=[0.99984 1.0013]  TsBlock=0
      settings: SourceProductBaseCode=PS
  Diesel Engine Governor : spsDieselMotorModel/Diesel Engine Governor  K=29  Tr=[0.01 0.02 0.2]  Ta=[0.25 0.009 0.0384]  Tlim=[0 1.1]  Td=0.024  Pm0=0.050008
      settings: SourceProductBaseCode=PS
  Generator Measures : Subsystem
  Ground : Ground
  Selected Measurements : Subsystem
  Synchronous Machine : spsSynchronousMachinepuStandardLib/Synchronous Machine pu Standard  PresetModel=No  MechanicalLoad=Mechanical power Pm  ShowDetailedParameters=on  RotorType=Salient-pole  Units=per unit standard parameters  MeasurementBus=off  NominalParameters=[ Pn Vn Fn]  Reactances1=[ 1.81, 0.3, 0.23, 1.76, 0.65, 0.25, 0.15 ]  Reactances2="[ 1.305, 0.296, 0.252, 0.474,  0.243,  0.18 ]"  dAxisTimeConstants=Open-circuit  qAxisTimeConstants=Short-circuit  TimeConstants1="[ 4.4849  0.0681  0.1  ]"  TimeConstants2=[ 8.0, 0.03, 1.0, 0.07 ]  TimeConstants3="[  4.49  0.0681  0.0513  ]"  TimeConstants4=[ 8.0, 0.03, 0.3371, 0.0295 ]  TimeConstants5=[ 1.01, 0.053, 0.1 ]  TimeConstants6=[ 1.3201, 0.023, 1.0, 0.07 ]  TimeConstants7=[0.012 0.003 0.003]  TimeConstants8=[ 1.3201, 0.0231, 0.3371, 0.0295 ]  StatorResistance=0.003  Mechanical=[3.7 0 1 ]  PolePairs=20  InitialConditions=[0 -88.646 0.0500078 0.0500078 0.0500078 -0.0038635 -120.004 119.996 1.00126]  SetSaturation=off  Saturation=[0.6404,0.7127,0.8441,0.9214,0.9956,1.082,1.19,1.316,1.457;0.7,0.7698,0.8872,0.9466,0.9969,1.046,1.1,1.151,1.201]  LoadFlowParameters=[1,0,0,0,0]  TsPowergui=0  TsBlock=-1  IterativeModel=Trapezoidal non iterative  IterativeDiscreteModel=Trapezoidal non iterative  BusType=PQ  Pref=Pn*P0  Qref=0  Qmin=-inf  Qmax=inf  PLF=0  QLF=0
      settings: SourceProductBaseCode=PS
  A : PMIOPort  Side=Right
  B : PMIOPort  Port=2  Side=Right
  C : PMIOPort  Port=3  Side=Right
  m : Outport  VectorParamsAs1DForOutWhenUnconnected=off
  wires:
  Selected Measurements/1(sm) -> m/1
  Generator Measures/1(Ifd) -> AC1A Excitation System/3
  Generator Measures/2(Vt) -> AC1A Excitation System/2
  Generator Measures/3(wm) -> Diesel Engine Governor/2
  Ground/1 -> AC1A Excitation System/4
  Synchronous Machine/1 -> Selected Measurements/1(m), Generator Measures/1(m)
  Vref (pu)/1 -> AC1A Excitation System/1
  AC1A Excitation System/1 -> Synchronous Machine/2
  Diesel Engine Governor/1 -> Synchronous Machine/1
  wref (pu)/1 -> Diesel Engine Governor/1
  connections:
  Synchronous Machine/RConn2 -- B/RConn1
  Synchronous Machine/RConn3 -- C/RConn1
  Synchronous Machine/RConn1 -- A/RConn1

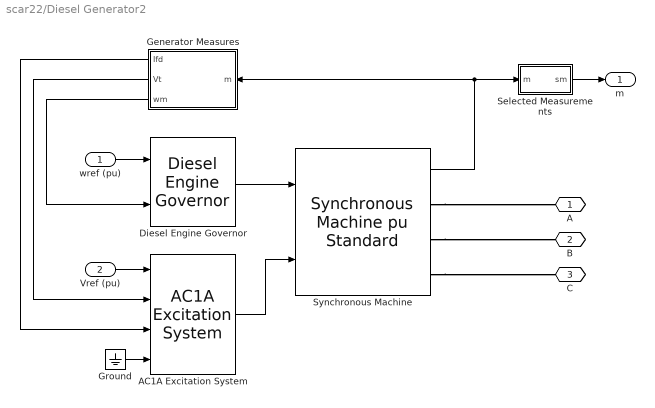
== system scar22/Diesel Generator2 ==
  wref (pu) : Inport
  Vref (pu) : Inport  Port=2
  AC1A Excitation System : spsAC1AExcitationSystemLib/AC1A Excitation System  Tr=20e-3  KaTa=[400 0.02]  VAminmax=[-14.5 14.5]  VRminmax=[-5.43 6.03]  KfTf=[0.03 1.0]  TbTc=[0 0]  KeTe=[1.0 0.80]  Ve12=[4.18 3.14]  SeVe12=[0.10 0.03]  Kd=0.38  Kc=0.20  v0=[0.99984 1.0013]  TsBlock=0
      settings: SourceProductBaseCode=PS
  Diesel Engine Governor : spsDieselMotorModel/Diesel Engine Governor  K=29  Tr=[0.01 0.02 0.2]  Ta=[0.25 0.009 0.0384]  Tlim=[0 1.1]  Td=0.024  Pm0=0.050008
      settings: SourceProductBaseCode=PS
  Generator Measures : Subsystem
  Ground : Ground
  Selected Measurements : Subsystem
  Synchronous Machine : spsSynchronousMachinepuStandardLib/Synchronous Machine pu Standard  PresetModel=No  MechanicalLoad=Mechanical power Pm  ShowDetailedParameters=on  RotorType=Salient-pole  Units=per unit standard parameters  MeasurementBus=off  NominalParameters=[ Pn Vn Fn]  Reactances1=[ 1.81, 0.3, 0.23, 1.76, 0.65, 0.25, 0.15 ]  Reactances2="[ 1.305, 0.296, 0.252, 0.474,  0.243,  0.18 ]"  dAxisTimeConstants=Open-circuit  qAxisTimeConstants=Short-circuit  TimeConstants1="[ 4.4849  0.0681  0.1  ]"  TimeConstants2=[ 8.0, 0.03, 1.0, 0.07 ]  TimeConstants3="[  4.49  0.0681  0.0513  ]"  TimeConstants4=[ 8.0, 0.03, 0.3371, 0.0295 ]  TimeConstants5=[ 1.01, 0.053, 0.1 ]  TimeConstants6=[ 1.3201, 0.023, 1.0, 0.07 ]  TimeConstants7=[0.012 0.003 0.003]  TimeConstants8=[ 1.3201, 0.0231, 0.3371, 0.0295 ]  StatorResistance=0.003  Mechanical=[3.7 0 1 ]  PolePairs=20  InitialConditions=[0 -88.646 0.0500078 0.0500078 0.0500078 -0.0038635 -120.004 119.996 1.00126]  SetSaturation=off  Saturation=[0.6404,0.7127,0.8441,0.9214,0.9956,1.082,1.19,1.316,1.457;0.7,0.7698,0.8872,0.9466,0.9969,1.046,1.1,1.151,1.201]  LoadFlowParameters=[1,0,0,0,0]  TsPowergui=0  TsBlock=-1  IterativeModel=Trapezoidal non iterative  IterativeDiscreteModel=Trapezoidal non iterative  BusType=PQ  Pref=Pn*P0  Qref=0  Qmin=-inf  Qmax=inf  PLF=0  QLF=0
      settings: SourceProductBaseCode=PS
  A : PMIOPort  Side=Right
  B : PMIOPort  Port=2  Side=Right
  C : PMIOPort  Port=3  Side=Right
  m : Outport  VectorParamsAs1DForOutWhenUnconnected=off
  wires:
  Selected Measurements/1(sm) -> m/1
  Generator Measures/1(Ifd) -> AC1A Excitation System/3
  Generator Measures/2(Vt) -> AC1A Excitation System/2
  Generator Measures/3(wm) -> Diesel Engine Governor/2
  Ground/1 -> AC1A Excitation System/4
  Synchronous Machine/1 -> Selected Measurements/1(m), Generator Measures/1(m)
  Vref (pu)/1 -> AC1A Excitation System/1
  AC1A Excitation System/1 -> Synchronous Machine/2
  Diesel Engine Governor/1 -> Synchronous Machine/1
  wref (pu)/1 -> Diesel Engine Governor/1
  connections:
  Synchronous Machine/RConn2 -- B/RConn1
  Synchronous Machine/RConn3 -- C/RConn1
  Synchronous Machine/RConn1 -- A/RConn1

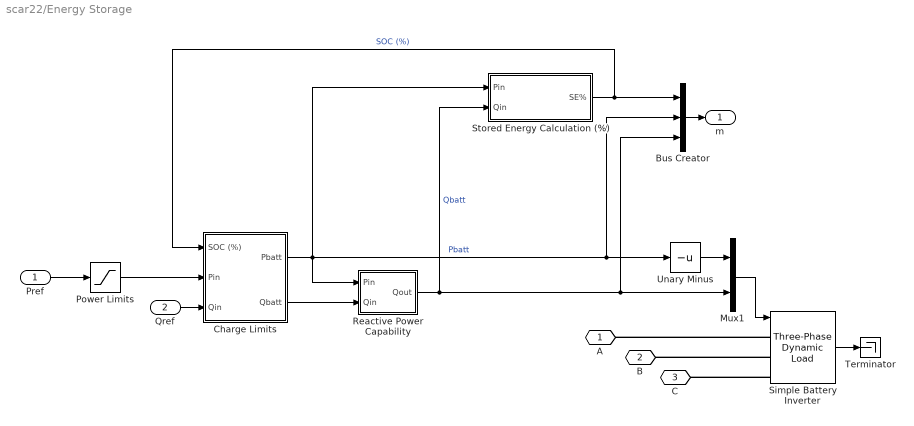
== system scar22/Energy Storage ==
  Pref : Inport
  Qref : Inport  Port=2
  Bus Creator : BusCreator  Inputs=3
  Charge Limits : Subsystem
  Mux1 : Mux  Inputs=2
  Power Limits : Saturate  UpperLimit=Pnom  LowerLimit=-Pnom
  Reactive Power Capability : Subsystem
  Simple Battery Inverter : spsThreePhaseDynamicLoadLib/Three-Phase Dynamic Load  NominalVoltage=[Vn Fn]  ActiveReactivePowers=[-500000 -3.38813e-13]  PositiveSequence=[0.999844 -0.0038635]  ExternalControl=on  NpNq=[1.3 2]  TimeConstants="[0  0  0  0]"  MinimumVoltage=0.7  Tfilter=1e-2  LoadFlowParameters=[4,0,0,0,0]
      settings: SourceProductBaseCode=PS
  Stored Energy Calculation (%) : Subsystem
  Terminator : Terminator
  Unary Minus : UnaryMinus
  A : PMIOPort  Side=Right
  B : PMIOPort  Port=2  Side=Right
  C : PMIOPort  Port=3  Side=Right
  m : Outport  VectorParamsAs1DForOutWhenUnconnected=off
  wires:
  Charge Limits/2(Qbatt) -> Reactive Power Capability/2(Qin)
  Qref/1 -> Charge Limits/3(Qin)
  Power Limits/1 -> Charge Limits/2(Pin)
  Charge Limits/1(Pbatt) -> Reactive Power Capability/1(Pin), Unary Minus/1, Bus Creator/2, Stored Energy Calculation (%)/1(Pin)  "Pbatt"
  Stored Energy Calculation (%)/1(SE%) -> Bus Creator/1, Charge Limits/1(SOC (%))  "SOC (%)"
  Bus Creator/1 -> m/1
  Pref/1 -> Power Limits/1
  Reactive Power Capability/1(Qout) -> Mux1/2, Bus Creator/3, Stored Energy Calculation (%)/2(Qin)  "Qbatt"
  Simple Battery Inverter/1 -> Terminator/1
  Mux1/1 -> Simple Battery Inverter/1
  Unary Minus/1 -> Mux1/1
  connections:
  Simple Battery Inverter/LConn1 -- A/RConn1
  Simple Battery Inverter/LConn3 -- C/RConn1
  Simple Battery Inverter/LConn2 -- B/RConn1

== system scar22/Phasor Sequence Analyzer ==
  Vabc : Inport
  Sequence Analyzer (Phasor) : spsSequenceAnalyzerPhasorLib/Sequence Analyzer (Phasor)  seq=Positive
      settings: SourceProductBaseCode=PS
  Terminator : Terminator
  Vrms : Outport  VectorParamsAs1DForOutWhenUnconnected=off
  wires:
  Sequence Analyzer (Phasor)/1 -> Vrms/1
  Vabc/1 -> Sequence Analyzer (Phasor)/1
  Sequence Analyzer (Phasor)/2 -> Terminator/1

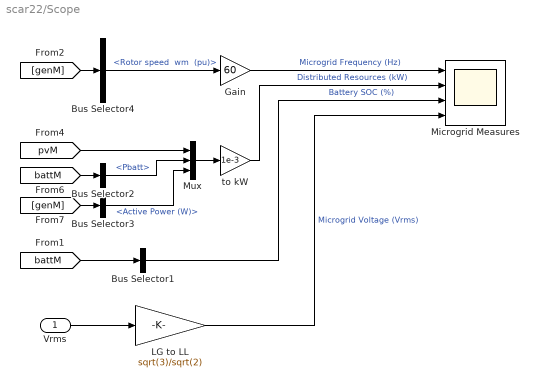
== system scar22/Scope ==
  Vrms : Inport
  Bus Selector1 : BusSelector  OutputSignals=SOC (%)  OutputAsBus=on
  Bus Selector2 : BusSelector  OutputSignals=Pbatt
  Bus Selector3 : BusSelector  OutputSignals=Active Power (W)
  Bus Selector4 : BusSelector  OutputSignals="Rotor speed  wm  (pu)"
  Gain : Gain  Gain=60
  LG to LL : Gain  Gain=sqrt(3)/sqrt(2)
  Microgrid Measures : Scope  NumInputPorts=4
  Mux : Mux  Inputs=3
  to kW : Gain  Gain=1e-3
  wires:
  Bus Selector3/1 -> Mux/3  "<Active Power (W)>"
  to kW/1 -> Microgrid Measures/2  "Distributed Resources (kW)"
  Bus Selector4/1 -> Gain/1  "<Rotor speed  wm  (pu)>"
  [genM] -> Bus Selector4/1
  Gain/1 -> Microgrid Measures/1  "Microgrid Frequency (Hz)"
  Bus Selector1/1 -> Microgrid Measures/3  "Battery SOC (%)"
  [battM] -> Bus Selector1/1
  [genM] -> Bus Selector3/1
  [battM] -> Bus Selector2/1
  Bus Selector2/1 -> Mux/2  "<Pbatt>"
  [pvM] -> Mux/1
  Mux/1 -> to kW/1
  LG to LL/1 -> Microgrid Measures/4  "Microgrid Voltage (Vrms)"
  Vrms/1 -> LG to LL/1

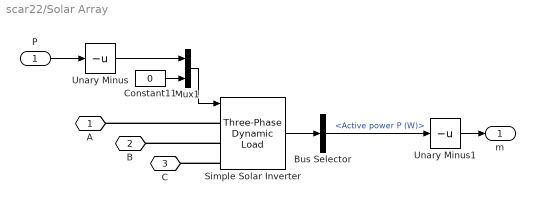
== system scar22/Solar Array ==
  P : Inport
  Bus Selector : BusSelector  OutputSignals=Active power P (W)
  Constant11 : Constant  Value=0
  Mux1 : Mux  Inputs=2
  Simple Solar Inverter : spsThreePhaseDynamicLoadLib/Three-Phase Dynamic Load  NominalVoltage=[Vn Fn]  ActiveReactivePowers=[-250000 -3.38813e-13]  PositiveSequence=[0.999844 -0.0038635]  ExternalControl=on  NpNq=[1.3 2]  TimeConstants="[0  0  0  0]"  MinimumVoltage=0.7  Tfilter=1e-2  LoadFlowParameters=[4,0,0,0,0]
      settings: SourceProductBaseCode=PS
  Unary Minus : UnaryMinus
  Unary Minus1 : UnaryMinus
  A : PMIOPort  Side=Right
  B : PMIOPort  Port=2  Side=Right
  C : PMIOPort  Port=3  Side=Right
  m : Outport  VectorParamsAs1DForOutWhenUnconnected=off
  wires:
  P/1 -> Unary Minus/1
  Unary Minus/1 -> Mux1/1
  Mux1/1 -> Simple Solar Inverter/1
  Constant11/1 -> Mux1/2
  Simple Solar Inverter/1 -> Bus Selector/1
  Bus Selector/1 -> Unary Minus1/1  "<Active power P (W)>"
  Unary Minus1/1 -> m/1
  connections:
  Simple Solar Inverter/LConn2 -- B/RConn1
  Simple Solar Inverter/LConn3 -- C/RConn1
  Simple Solar Inverter/LConn1 -- A/RConn1

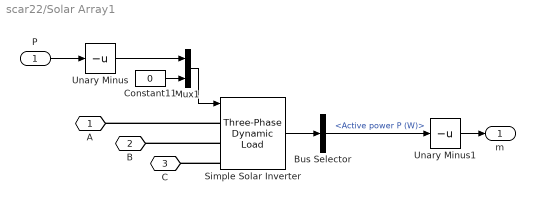
== system scar22/Solar Array1 ==
  P : Inport
  Bus Selector : BusSelector  OutputSignals=Active power P (W)
  Constant11 : Constant  Value=0
  Mux1 : Mux  Inputs=2
  Simple Solar Inverter : spsThreePhaseDynamicLoadLib/Three-Phase Dynamic Load  NominalVoltage=[Vn Fn]  ActiveReactivePowers=[-250000 -3.38813e-13]  PositiveSequence=[0.999844 -0.0038635]  ExternalControl=on  NpNq=[1.3 2]  TimeConstants="[0  0  0  0]"  MinimumVoltage=0.7  Tfilter=1e-2  LoadFlowParameters=[4,0,0,0,0]
      settings: SourceProductBaseCode=PS
  Unary Minus : UnaryMinus
  Unary Minus1 : UnaryMinus
  A : PMIOPort  Side=Right
  B : PMIOPort  Port=2  Side=Right
  C : PMIOPort  Port=3  Side=Right
  m : Outport  VectorParamsAs1DForOutWhenUnconnected=off
  wires:
  Unary Minus1/1 -> m/1
  Bus Selector/1 -> Unary Minus1/1  "<Active power P (W)>"
  Simple Solar Inverter/1 -> Bus Selector/1
  Constant11/1 -> Mux1/2
  Mux1/1 -> Simple Solar Inverter/1
  Unary Minus/1 -> Mux1/1
  P/1 -> Unary Minus/1
  connections:
  Simple Solar Inverter/LConn1 -- A/RConn1
  Simple Solar Inverter/LConn3 -- C/RConn1
  Simple Solar Inverter/LConn2 -- B/RConn1

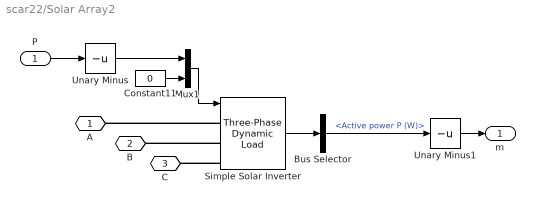
== system scar22/Solar Array2 ==
  P : Inport
  Bus Selector : BusSelector  OutputSignals=Active power P (W)
  Constant11 : Constant  Value=0
  Mux1 : Mux  Inputs=2
  Simple Solar Inverter : spsThreePhaseDynamicLoadLib/Three-Phase Dynamic Load  NominalVoltage=[Vn Fn]  ActiveReactivePowers=[-250000 -3.38813e-13]  PositiveSequence=[0.999844 -0.0038635]  ExternalControl=on  NpNq=[1.3 2]  TimeConstants="[0  0  0  0]"  MinimumVoltage=0.7  Tfilter=1e-2  LoadFlowParameters=[4,0,0,0,0]
      settings: SourceProductBaseCode=PS
  Unary Minus : UnaryMinus
  Unary Minus1 : UnaryMinus
  A : PMIOPort  Side=Right
  B : PMIOPort  Port=2  Side=Right
  C : PMIOPort  Port=3  Side=Right
  m : Outport  VectorParamsAs1DForOutWhenUnconnected=off
  wires:
  P/1 -> Unary Minus/1
  Unary Minus/1 -> Mux1/1
  Mux1/1 -> Simple Solar Inverter/1
  Constant11/1 -> Mux1/2
  Simple Solar Inverter/1 -> Bus Selector/1
  Bus Selector/1 -> Unary Minus1/1  "<Active power P (W)>"
  Unary Minus1/1 -> m/1
  connections:
  Simple Solar Inverter/LConn2 -- B/RConn1
  Simple Solar Inverter/LConn3 -- C/RConn1
  Simple Solar Inverter/LConn1 -- A/RConn1

== system scar22/Transmission Line1 ==
  Three-Phase Series RL Branch : spsThreePhaseSeriesRLCBranchLib/Three-Phase Series RLC Branch  LConnTagsString=A|B|C  RConnTagsString=A|B|C  BranchType=RL  Resistance=R*Length  Inductance=L*Length  Capacitance=1e-6  Measurements=None
  A : PMIOPort  Side=Left
  B : PMIOPort  Port=2  Side=Left
  C : PMIOPort  Port=3  Side=Left
  a : PMIOPort  Port=4  Side=Right
  b : PMIOPort  Port=5  Side=Right
  c : PMIOPort  Port=6  Side=Right
  connections:
  B/RConn1 -- Three-Phase Series RL Branch/LConn2
  C/RConn1 -- Three-Phase Series RL Branch/LConn3
  Three-Phase Series RL Branch/RConn2 -- b/RConn1
  A/RConn1 -- Three-Phase Series RL Branch/LConn1
  Three-Phase Series RL Branch/RConn3 -- c/RConn1
  Three-Phase Series RL Branch/RConn1 -- a/RConn1
